simulink model "q3"  (R2023a)
settings: Solver=VariableStepAuto  StartTime=0.0  StopTime=10.0  RelTol=1e-3
libraries: commdigbbndam3 x2, commchan3 x1, commsink2 x1, commrandsrc3 x1
settings Model: Creator=giri0  LastModifiedBy=giri0

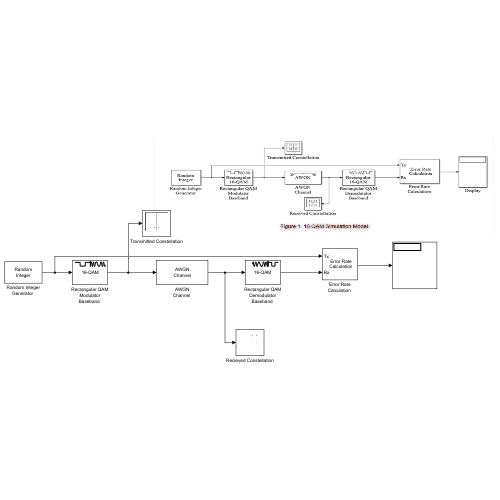
[thumbnail: Simulink's stored preview of the top-level diagram]
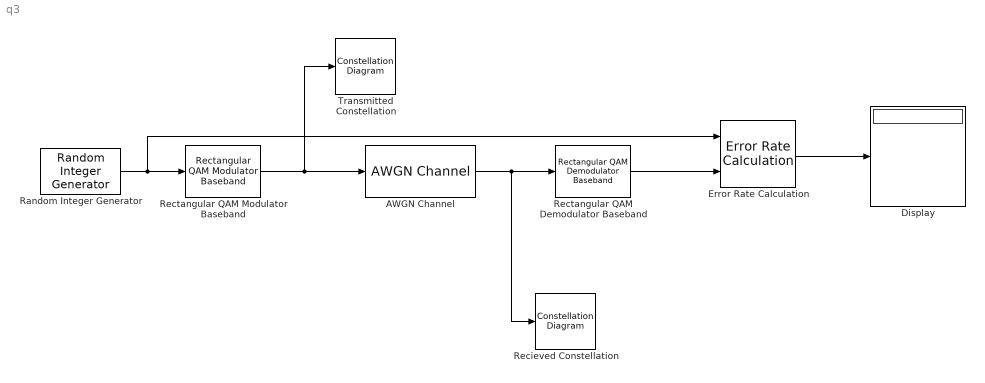
== system q3 ==
  "AWGN Channel " : commchan3/AWGN Channel  LegacyMode=off  NoiseMethod="Signal to noise ratio  (Eb/No)"  noiseMode="Signal to noise ratio  (SNR)"  EbNo=1e-6  EsNo=10  SNR=10  BitsPerSymbol=4  SignalPower=1  SamplesPerSymbol=1  SymbolPeriod=1  VarianceSource=Parameter  Variance=1  RandomStream=Global stream  Seed=67  SimulateUsing=Code generation
  Display : Display
  "Error Rate Calculation " : commsink2/Error Rate Calculation  N=0  st_delay=0  cp_mode=Entire frame  subframe=[]  PMode=Port  WsName=ErrorVec  RsMode2=off  stop=off  numErr=100  maxBits=1e6
  "Random Integer Generator " : commrandsrc3/Random Integer Generator  SetSize=8  SeedSource=Auto  Seed=0  SampleTime=1e-6  SamplesPerFrame=1024  OutputDataType=double  SimulateUsing=Interpreted execution
  Recieved Constellation : ConstellationDiagram
  "Rectangular QAM Demodulator Baseband " : commdigbbndam3/Rectangular QAM Demodulator Baseband  M=16  OutType=Integer  DecType=Hard decision  VarSource=Dialog  Variance=1  Dec=Gray  Mapping=[0:15]  PowType=Peak Power  MinDist=2  AvgPow=1  PeakPow=1  Ph=0  outDtype1=Inherit via internal rule  outDtype2=Inherit via internal rule  derotateFactorWordLen=16  derotateFactorDataTypeStr=Inherit: Same word length as input  derotateFactorLastDataTypeStr=Inherit: Same word length as input  denormFactorWordLen=16  denormFactorDataTypeStr=Inherit: Same word length as input  denormFactorLastDataTypeStr=Inherit: Same word length as input  prodOutWordLen=32  prodOutOverflowMode=Wrap  prodOutRoundingMode=Floor  prodOutOvFlMode=off  prodOutOvFlModeLastStrValue=off  sumWordLen=32
  "Rectangular QAM Modulator Baseband " : commdigbbndam3/Rectangular QAM Modulator Baseband  M=16  InType=Integer  Enc=Gray  Mapping=[0:15]  PowType=Peak Power  MinDist=2  AvgPow=1  PeakPow=1  Ph=0  outDtype=double  outWordLen=16  outUDDataType=sfix(16)  outFracLenMode=Best precision  outFracLen=15  outDataTypeStr=double  outLastDataTypeStr=double
      settings: LibrarySourceBlock=|
      | commhdldigbbndam/Rectangular QAM
      | Modulator
      | Baseband
  Transmitted Constellation : ConstellationDiagram  WindowPosition=[382.000000,84.000000,600.000000,600.000000,]  ScopeFrameLocation=window
  wires:
  "Rectangular QAM Demodulator Baseband "/1 -> "Error Rate Calculation "/2
  "Random Integer Generator "/1 -> "Error Rate Calculation "/1, "Rectangular QAM Modulator Baseband "/1
  "AWGN Channel "/1 -> Recieved Constellation/1, "Rectangular QAM Demodulator Baseband "/1
  "Rectangular QAM Modulator Baseband "/1 -> Transmitted Constellation/1, "AWGN Channel "/1
  "Error Rate Calculation "/1 -> Display/1
